simulink model "pct"  (Simulink 10.0)
settings: Solver=FixedStepDiscrete  StartTime=0.0  StopTime=16000.0  RelTol=1e-3
settings Model: Creator=fox3mue  LastModifiedBy=bhisma
settings SolverCC: AutoInsertRateTranBlk=on
settings DataIOCC: LimitDataPoints=on  SignalLoggingSaveFormat=ModelDataLogs
settings OptimizationCC: BlockReduction=off  ConditionallyExecuteInputs=off  ExpressionDepthLimit=2147483647
settings DebuggingCC: SolverPrmCheckMsg=warning  MultiTaskCondExecSysMsg=warning  MultiTaskRateTransMsg=warning  FcnCallInpInsideContextMsg=warning  StateNameClashWarn=warning
settings GRTTargetCC: GeneratePreprocessorConditionals=Disable all
settings ConfigComp: CovExternalEMLEnable=off  CovSFcnEnable=off

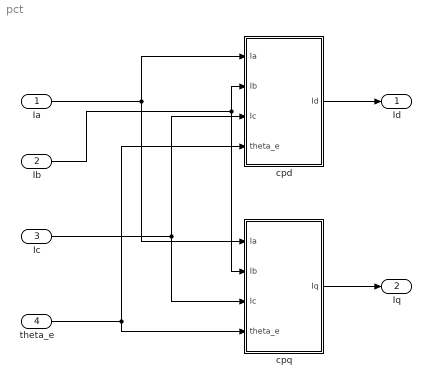
== system pct ==
  Ia : Inport
  Ib : Inport  Port=2
  Ic : Inport  Port=3
  theta_e : Inport  Port=4
  cpd : Subsystem
  cpq : Subsystem
  Id : Outport
  Iq : Outport  Port=2
  wires:
  theta_e/1 -> cpd/4(theta_e), cpq/4(theta_e)
  Ia/1 -> cpd/1(Ia), cpq/1(Ia)
  Ib/1 -> cpd/2(Ib), cpq/2(Ib)
  Ic/1 -> cpd/3(Ic), cpq/3(Ic)
  cpd/1(Id) -> Id/1
  cpq/1(Iq) -> Iq/1

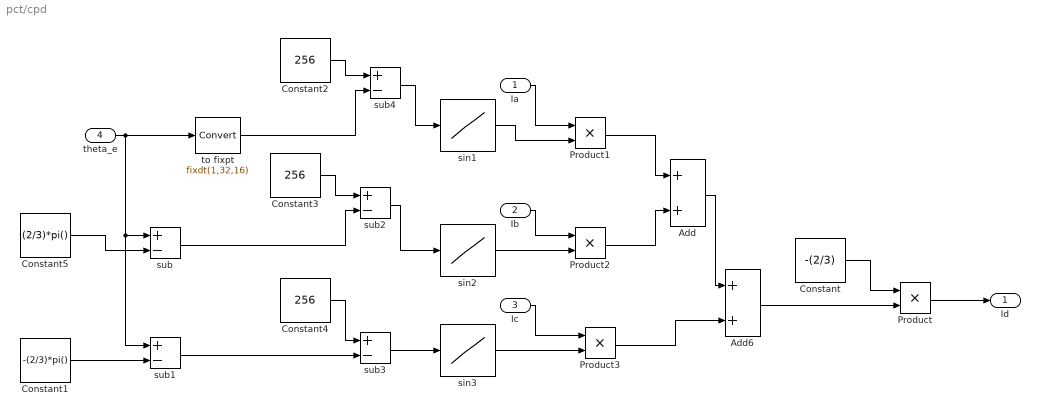
== system pct/cpd ==
  Ia : Inport
  Ib : Inport  Port=2
  Ic : Inport  Port=3
  theta_e : Inport  Port=4
  Add : Sum  AccumDataTypeStr=fixdt(1,64,43)  OutDataTypeStr=fixdt(1,64,43)
  Add6 : Sum  AccumDataTypeStr=fixdt(1,64,43)  OutDataTypeStr=fixdt(1,64,43)
  Constant : Constant  Value=-(2/3)  OutDataTypeStr=Inherit: Inherit via back propagation
  Constant1 : Constant  Value=-(2/3)*pi()  OutDataTypeStr=Inherit: Inherit via back propagation
  Constant2 : Constant  Value=256  OutDataTypeStr=Inherit: Inherit via back propagation
  Constant3 : Constant  Value=256  OutDataTypeStr=Inherit: Inherit via back propagation
  Constant4 : Constant  Value=256  OutDataTypeStr=Inherit: Inherit via back propagation
  Constant5 : Constant  Value=(2/3)*pi()  OutDataTypeStr=Inherit: Inherit via back propagation
  Product{,1..3} (4 alike) : Product  OutDataTypeStr=fixdt(1,48,43)  RndMeth=Zero
  sin1 : Lookup_n-D  NumberOfTableDimensions=1  BreakpointsForDimension1=[0:1024]  IndexSearchMethod=Evenly spaced points  BeginIndexSearchUsingPreviousIndexResult=on  Table=sin((0:1024))'  ExtrapMethod=Clip  DiagnosticForOutOfRangeInput=Warning  RemoveProtectionInput=on  UseLastTableValue=on  OutDataTypeStr=fixdt(1,16,15)  InputSameDT=on
  sin2 : Lookup_n-D  NumberOfTableDimensions=1  BreakpointsForDimension1=[0:1024]  IndexSearchMethod=Evenly spaced points  BeginIndexSearchUsingPreviousIndexResult=on  Table=sin((0:1024))'  ExtrapMethod=Clip  DiagnosticForOutOfRangeInput=Warning  RemoveProtectionInput=on  UseLastTableValue=on  OutDataTypeStr=fixdt(1,16,15)  InputSameDT=on
  sin3 : Lookup_n-D  NumberOfTableDimensions=1  BreakpointsForDimension1=[0:1024]  IndexSearchMethod=Evenly spaced points  BeginIndexSearchUsingPreviousIndexResult=on  Table=sin((0:1024))'  ExtrapMethod=Clip  DiagnosticForOutOfRangeInput=Warning  RemoveProtectionInput=on  UseLastTableValue=on  OutDataTypeStr=fixdt(1,16,15)  InputSameDT=on
  sub{,1..4} (5 alike) : Sum  Inputs=+-  AccumDataTypeStr=fixdt(1,32,16)  OutDataTypeStr=fixdt(1,32,16)
  "to fixpt " : DataTypeConversion  OutDataTypeStr=fixdt(1,32,16)
  Id : Outport
  wires:
  Constant/1 -> Product/1
  Product/1 -> Id/1
  Product1/1 -> Add/1
  Product2/1 -> Add/2
  Ia/1 -> Product1/1
  Ib/1 -> Product2/1
  Ic/1 -> Product3/1
  theta_e/1 -> sub1/1, sub/1, "to fixpt "/1
  Constant1/1 -> sub1/2
  sin1/1 -> Product1/2
  sub/1 -> sub2/2
  sub1/1 -> sub3/2
  Constant2/1 -> sub4/1
  Constant3/1 -> sub2/1
  Constant4/1 -> sub3/1
  "to fixpt "/1 -> sub4/2
  sub4/1 -> sin1/1
  sub2/1 -> sin2/1
  Product3/1 -> Add6/2
  Add/1 -> Add6/1
  Add6/1 -> Product/2
  sin2/1 -> Product2/2
  sub3/1 -> sin3/1
  sin3/1 -> Product3/2
  Constant5/1 -> sub/2

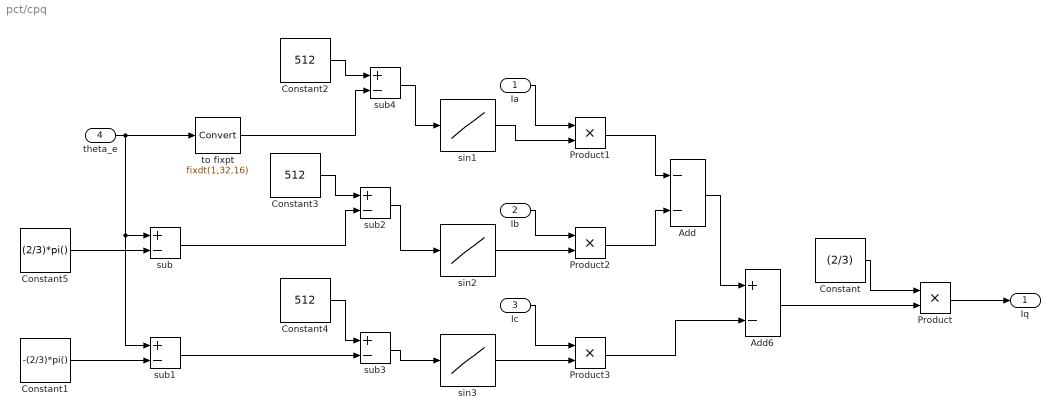
== system pct/cpq ==
  Ia : Inport
  Ib : Inport  Port=2
  Ic : Inport  Port=3
  theta_e : Inport  Port=4
  Add : Sum  Inputs=--  AccumDataTypeStr=fixdt(1,64,43)  OutDataTypeStr=fixdt(1,64,43)
  Add6 : Sum  Inputs=+-  AccumDataTypeStr=fixdt(1,64,43)  OutDataTypeStr=fixdt(1,64,43)
  Constant : Constant  Value=(2/3)  OutDataTypeStr=Inherit: Inherit via back propagation
  Constant1 : Constant  Value=-(2/3)*pi()  OutDataTypeStr=Inherit: Inherit via back propagation
  Constant2 : Constant  Value=512  OutDataTypeStr=Inherit: Inherit via back propagation
  Constant3 : Constant  Value=512  OutDataTypeStr=Inherit: Inherit via back propagation
  Constant4 : Constant  Value=512  OutDataTypeStr=Inherit: Inherit via back propagation
  Constant5 : Constant  Value=(2/3)*pi()  OutDataTypeStr=Inherit: Inherit via back propagation
  Product{,1..3} (4 alike) : Product  OutDataTypeStr=fixdt(1,48,43)  RndMeth=Zero
  sin1 : Lookup_n-D  NumberOfTableDimensions=1  BreakpointsForDimension1=[0:1024]  IndexSearchMethod=Evenly spaced points  BeginIndexSearchUsingPreviousIndexResult=on  Table=sin((0:1024))'  ExtrapMethod=Clip  DiagnosticForOutOfRangeInput=Warning  RemoveProtectionInput=on  UseLastTableValue=on  OutDataTypeStr=fixdt(1,16,15)  InputSameDT=on
  sin2 : Lookup_n-D  NumberOfTableDimensions=1  BreakpointsForDimension1=[0:1024]  IndexSearchMethod=Evenly spaced points  BeginIndexSearchUsingPreviousIndexResult=on  Table=sin((0:1024))'  ExtrapMethod=Clip  DiagnosticForOutOfRangeInput=Warning  RemoveProtectionInput=on  UseLastTableValue=on  OutDataTypeStr=fixdt(1,16,15)  InputSameDT=on
  sin3 : Lookup_n-D  NumberOfTableDimensions=1  BreakpointsForDimension1=[0:1024]  IndexSearchMethod=Evenly spaced points  BeginIndexSearchUsingPreviousIndexResult=on  Table=sin((0:1024))'  ExtrapMethod=Clip  DiagnosticForOutOfRangeInput=Warning  RemoveProtectionInput=on  UseLastTableValue=on  OutDataTypeStr=fixdt(1,16,15)  InputSameDT=on
  sub{,1..4} (5 alike) : Sum  Inputs=+-  AccumDataTypeStr=fixdt(1,32,16)  OutDataTypeStr=fixdt(1,32,16)
  "to fixpt " : DataTypeConversion  OutDataTypeStr=fixdt(1,32,16)
  Iq : Outport
  wires:
  Constant/1 -> Product/1
  Product/1 -> Iq/1
  Product1/1 -> Add/1
  Product2/1 -> Add/2
  Ia/1 -> Product1/1
  Ib/1 -> Product2/1
  Ic/1 -> Product3/1
  theta_e/1 -> sub1/1, sub/1, "to fixpt "/1
  Constant1/1 -> sub1/2
  sin1/1 -> Product1/2
  sub/1 -> sub2/2
  sub1/1 -> sub3/2
  Constant2/1 -> sub4/1
  Constant3/1 -> sub2/1
  Constant4/1 -> sub3/1
  "to fixpt "/1 -> sub4/2
  sub4/1 -> sin1/1
  sub2/1 -> sin2/1
  Product3/1 -> Add6/2
  Add/1 -> Add6/1
  Add6/1 -> Product/2
  sin2/1 -> Product2/2
  sub3/1 -> sin3/1
  sin3/1 -> Product3/2
  Constant5/1 -> sub/2
